simulink model "zad6simulink"  (R2023a)
settings: Solver=VariableStepAuto  StartTime=0.0  StopTime=100  RelTol=1e-3
values from neighbouring files (symbols this model uses):
  Gz = c2d(Gs,T,'zoh')    [zad1.m]
  Kpor = acker(A,B,bieguny)    [zad4.m]
  L = [double(lx.l1); double(lx.l2); double(lx.l3)]    [zad6.m]
  T = 0.5    [zad1.m]    (also in zad4.mat)
settings Model: Creator=pkutyl  LastModifiedBy=pkutyl

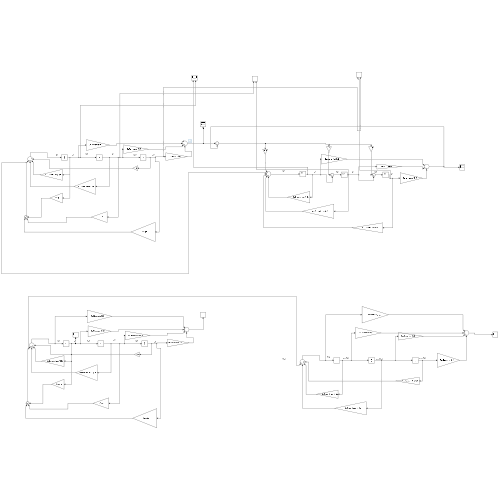
[thumbnail: Simulink's stored preview of the top-level diagram]
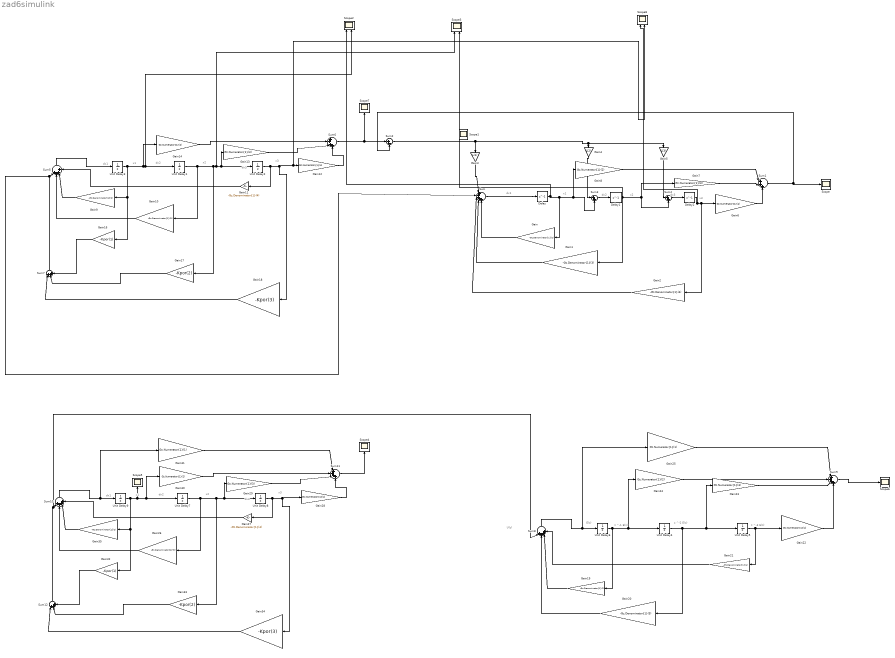
== system zad6simulink ==
  note: x3
  note: dx3
  note: x2
  note: dx2
  note: x1
  note: dx1
  note: x2
  note: dx1
  note: x1
  note: dx2
  note: dx3
  note: x3
  note: U(z)
  note: z ^-3 E(z)
  note: z ^-2 E(z)
  note: z ^-1 E(z)
  note: E(z)
  note: dx1
  note: x1
  note: x3
  note: x2
  note: dx2
  note: dx3
  Delay : Delay  DelayLength=1  InitialCondition=0  SampleTime=T
  Delay1 : Delay  DelayLength=1  InitialCondition=0  SampleTime=T
  Delay2 : Delay  DelayLength=1  InitialCondition=0  SampleTime=T
  Gain{,9,19,35} (4 alike) : Gain  Gain=-Gz.Denominator{1}(2)
  Gain{1,10,20,26} (4 alike) : Gain  Gain=-Gz.Denominator{1}(3)
  Gain{2,11,21,27} (4 alike) : Gain  Gain=-Gz.Denominator{1}(4)
  Gain{6,12,22,28} (4 alike) : Gain  Gain=Gz.Numerator{1}(4)
  Gain{7,13,23,29} (4 alike) : Gain  Gain=Gz.Numerator{1}(3)
  Gain{8,14,24,30} (4 alike) : Gain  Gain=Gz.Numerator{1}(2)
  Gain16 : Gain  Gain=-Kpor(1)
  Gain17 : Gain  Gain=-Kpor(2)
  Gain18 : Gain  Gain=-Kpor(3)
  Gain25 : Gain  Gain=Gz.Numerator{1}(1)
  Gain3 : Gain  Gain=L(1)
  Gain31 : Gain  Gain=Gz.Numerator{1}(1)
  Gain32 : Gain  Gain=-Kpor(1)
  Gain33 : Gain  Gain=-Kpor(2)
  Gain34 : Gain  Gain=-Kpor(3)
  Gain4 : Gain  Gain=L(2)
  Gain5 : Gain  Gain=L(3)
  Scope{,1,4..7} (6 alike) : Scope
  Scope2 : Scope  NumInputPorts=2
  Scope3 : Scope  NumInputPorts=2
  Scope8 : Scope  NumInputPorts=2
  Sum : Sum  Inputs=|+++++
  Sum1 : Sum  Inputs=|+++
  Sum{5..6,8..11} (6 alike) : Sum  Inputs=|++++
  Sum12 : Sum  Inputs=|+++
  Sum2 : Sum  Inputs=|+-
  Sum3 : Sum  Inputs=|++
  Sum4 : Sum  Inputs=|++
  Sum7 : Sum  Inputs=|+++
  Unit Delay1 : UnitDelay  InitialCondition=1  SampleTime=T  HasFrameUpgradeWarning=on
  Unit Delay2 : UnitDelay  InitialCondition=-1  SampleTime=T  HasFrameUpgradeWarning=on
  Unit Delay3 : UnitDelay  InitialCondition=2  SampleTime=T  HasFrameUpgradeWarning=on
  Unit Delay4 : UnitDelay  InitialCondition=1  SampleTime=T  HasFrameUpgradeWarning=on
  Unit Delay5 : UnitDelay  InitialCondition=-1  SampleTime=T  HasFrameUpgradeWarning=on
  Unit Delay6 : UnitDelay  InitialCondition=2  SampleTime=T  HasFrameUpgradeWarning=on
  Unit Delay7 : UnitDelay  InitialCondition=1  SampleTime=T  HasFrameUpgradeWarning=on
  Unit Delay8 : UnitDelay  InitialCondition=-1  SampleTime=T  HasFrameUpgradeWarning=on
  Unit Delay9 : UnitDelay  InitialCondition=2  SampleTime=T  HasFrameUpgradeWarning=on
  wires:
  Delay/1 -> Gain/1, Sum3/2, Gain8/1, Scope2/1
  Delay1/1 -> Scope3/2, Gain7/1, Sum4/2, Gain1/1
  Sum/1 -> Delay/1
  Delay2/1 -> Scope8/1, Gain6/1, Gain2/1
  Gain/1 -> Sum/5
  Gain1/1 -> Sum/4
  Gain2/1 -> Sum/3
  Gain3/1 -> Sum/1
  Gain6/1 -> Sum1/3
  Gain7/1 -> Sum1/2
  Gain8/1 -> Sum1/1
  Sum2/1 -> Gain5/1, Gain4/1, Gain3/1
  Gain4/1 -> Sum3/1
  Sum3/1 -> Delay1/1
  Gain5/1 -> Sum4/1
  Sum4/1 -> Delay2/1
  Gain13/1 -> Sum6/3
  Sum5/1 -> Unit Delay3/1
  Gain10/1 -> Sum5/2
  Gain11/1 -> Sum5/4
  Unit Delay3/1 -> Gain16/1, Gain9/1, Scope2/2, Unit Delay1/1, Gain14/1
  Gain9/1 -> Sum5/3
  Unit Delay2/1 -> Gain18/1, Scope8/2, Gain12/1, Gain11/1
  Unit Delay1/1 -> Gain10/1, Gain17/1, Scope3/1, Gain13/1, Unit Delay2/1
  Gain12/1 -> Sum6/4
  Gain14/1 -> Sum6/2
  Gain17/1 -> Sum7/2
  Gain18/1 -> Sum7/1
  Gain16/1 -> Sum7/3
  Sum7/1 -> Sum5/1, Sum/2
  Sum6/1 -> Scope7/1, Sum2/1
  Sum1/1 -> Sum2/2, Scope/1
  Gain20/1 -> Sum8/2
  Unit Delay4/1 -> Gain20/1, Gain23/1, Unit Delay5/1
  Sum8/1 -> Unit Delay6/1, Gain25/1
  Sum12/1 -> Sum8/1, Sum10/1
  Gain19/1 -> Sum8/3
  Gain22/1 -> Sum9/4
  Gain21/1 -> Sum8/4
  Unit Delay6/1 -> Gain19/1, Gain24/1, Unit Delay4/1
  Gain23/1 -> Sum9/3
  Gain24/1 -> Sum9/2
  Unit Delay5/1 -> Gain21/1, Gain22/1
  Sum9/1 -> Scope6/1
  Gain25/1 -> Sum9/1
  Gain31/1 -> Sum11/1
  Sum11/1 -> Scope4/1
  Gain30/1 -> Sum11/2
  Gain32/1 -> Sum12/3
  Unit Delay7/1 -> Gain26/1, Gain33/1, Gain29/1, Unit Delay8/1
  Unit Delay8/1 -> Gain34/1, Gain28/1, Gain27/1
  Unit Delay9/1 -> Gain32/1, Gain35/1, Scope5/1, Gain30/1, Unit Delay7/1
  Gain28/1 -> Sum11/4
  Gain35/1 -> Sum10/3
  Gain34/1 -> Sum12/1
  Gain33/1 -> Sum12/2
  Gain26/1 -> Sum10/2
  Gain29/1 -> Sum11/3
  Sum10/1 -> Unit Delay9/1, Gain31/1
  Gain27/1 -> Sum10/4
